simulink model "motor_cal"  (R2022b)
settings: Solver=FixedStepAuto  StartTime=0.0  StopTime=12  RelTol=1e-3  EnableMultiTasking=on
undefined symbols (not defined in the file or in its folder): ODR
libraries: raspberrypiBasiclib x6, raspberrypiIMUsensorslib x2, simulink x1
settings Model: Creator=sjohnson  LastModifiedBy=sjohnson
settings SolverCC: PositivePriorityOrder=on
settings OptimizationCC: EnhancedBackFolding=on  PassReuseOutputArgsAs=Individual arguments  ZeroExternalMemoryAtStartup=off  ZeroInternalMemoryAtStartup=off  MaxStackSize=64  OptimizeBlockOrder=speed  DifferentSizesBufferReuse=on  OptimizationCustomize=off  EfficientTunableParamExpr=on
settings DebuggingCC: ParameterTunabilityLossMsg=error
settings HardwareCC: ProdBitPerPointer=32  ProdBitPerSizeT=32  ProdBitPerPtrDiffT=32  ProdLargestAtomicInteger=Long  ProdLargestAtomicFloat=Double  ProdWordSize=32  ProdLongLongMode=on  ProdHWDeviceType=ARM Compatible->ARM Cortex  UseEmbeddedCoderFeatures=off  UseSimulinkCoderFeatures=off
settings ModelReferenceCC: UpdateModelReferenceTargets=AssumeUpToDate
settings RTWCC: Description=Embedded Coder  SystemTargetFile=ert.tlc  HardwareBoard=Raspberry Pi  TLCOptions="-aInlineSetEventsForThisBaseRateFcn=TLC_FALSE -aSuppressMultiTaskScheduler=TLC_FALSE  -aRateBasedStepFcn=0"  TemplateMakefile=ert_default_tmf  Toolchain=GNU GCC Embedded Linux  BuildConfiguration=Faster Runs
settings CodeAppCC: ForceParamTrailComments=on  IgnoreCustomStorageClasses=off  OperatorAnnotations=on  SimulinkDataObjDesc=on  SFDataObjDesc=on  MangleLength=10  InsertBlockDesc=on
settings ERTTargetCC: SupportNonInlinedSFcns=on  SupportVariableSizeSignals=on  ExtModeTransport=2  ExtModeStaticAlloc=on  ExtModeMexFile=ext_xcp  ExtModeIntrfLevel=Level2 - Open

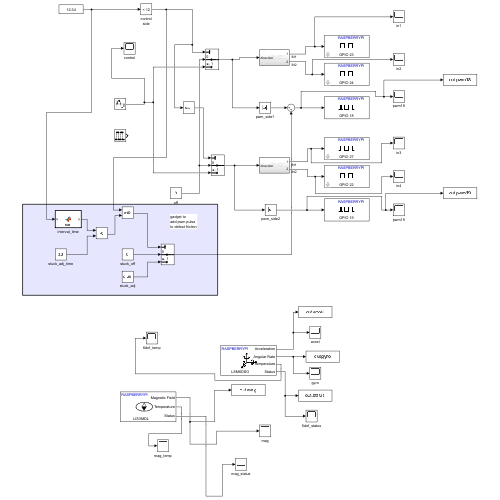
[thumbnail: Simulink's stored preview of the top-level diagram]
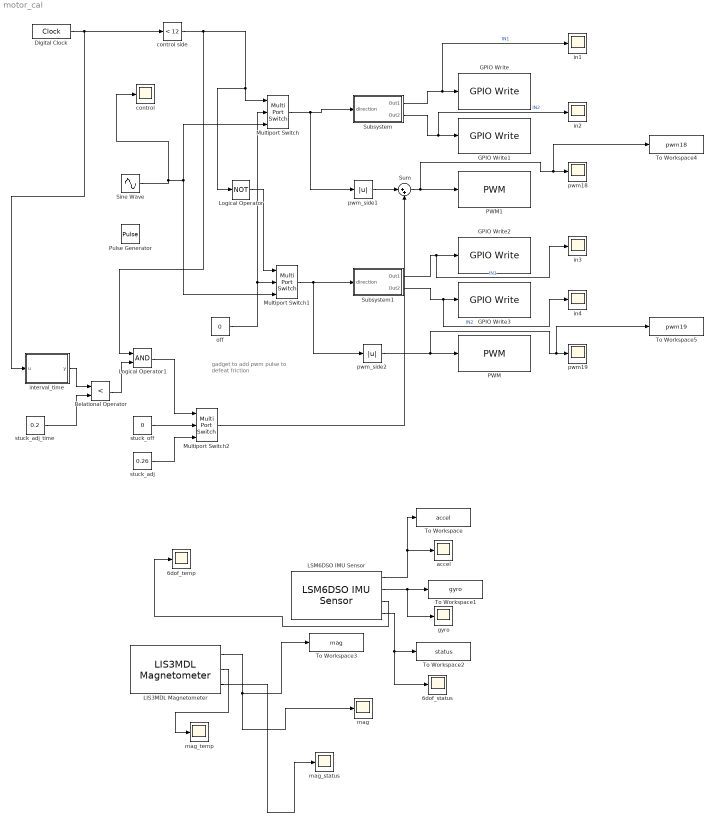
== system motor_cal ==
  note: gadget to
      | add pwm pulse
      | to defeat friction
  6dof_status : Scope
  6dof_temp : Scope
  Digital Clock : DigitalClock  SampleTime=.01
  GPIO Write : raspberrypiBasiclib/GPIO Write  board=Pi 4 Model B  gpio=23  direction=Output  blockPlatform=Raspberry Pi
  GPIO Write1 : raspberrypiBasiclib/GPIO Write  board=Pi 4 Model B  gpio=24  direction=Output  blockPlatform=Raspberry Pi
  GPIO Write2 : raspberrypiBasiclib/GPIO Write  board=Pi 4 Model B  gpio=27  direction=Output  blockPlatform=Raspberry Pi
  GPIO Write3 : raspberrypiBasiclib/GPIO Write  board=Pi 4 Model B  gpio=22  direction=Output  blockPlatform=Raspberry Pi
  LIS3MDL Magnetometer : raspberrypiIMUsensorslib/LIS3MDL Magnetometer  I2CModule=1  I2CAddress=0x1E  IsActiveMagnetometer=on  IsActiveTemperature=on  IsStatus=on  SampleTime=-1  MagnetometerRange=+/- 400 uT  MagnetometerODR=155 Hz
  LSM6DSO IMU Sensor : raspberrypiIMUsensorslib/LSM6DSO IMU Sensor  I2CModule=1  I2CAddress=0x6B  IsActiveAcceleration=on  IsActiveAngularRate=on  IsActiveTemperature=on  IsActiveStatus=on  IsActiveTimeStamp=off  SampleTime=-1  QueueSizeFactor=3  AccelerometerRange=+/- 2g  AccelerometerODR=104 Hz  AccelSelectCompositeFilter=No filter  AccelLPF2BW=ODR/4  AccelHPFBW=ODR/4  GyroscopeRange=125 dps  GyroscopeODR=104 Hz  EnableGyroHPF=off  GyroHPFBW=0.016 Hz  EnableGyroLPF=off  GyroLPFBWMode=0
  Logical Operator : Logic  Operator=NOT  Inputs=1  AllPortsSameDT=off  OutDataTypeStr=boolean
  Logical Operator1 : Logic  AllPortsSameDT=off  OutDataTypeStr=boolean
  Multiport Switch : MultiPortSwitch  DataPortOrder=Zero-based contiguous  Inputs=2  zeroidx=on  SaturateOnIntegerOverflow=off  InputSameDT=off
  Multiport Switch1 : MultiPortSwitch  DataPortOrder=Zero-based contiguous  Inputs=2  zeroidx=on  SaturateOnIntegerOverflow=off  InputSameDT=off
  Multiport Switch2 : MultiPortSwitch  DataPortOrder=Zero-based contiguous  Inputs=2  zeroidx=on  SaturateOnIntegerOverflow=off  InputSameDT=off
  PWM : raspberrypiBasiclib/PWM  board=Pi 4 Model B  Pin_=19  Frequency=50  blockPlatform=Raspberry Pi
  PWM1 : raspberrypiBasiclib/PWM  board=Pi 4 Model B  Pin_=18  Frequency=50  blockPlatform=Raspberry Pi
  Pulse Generator : DiscretePulseGenerator  Period=200  PulseWidth=50  SampleTime=0.01
  Relational Operator : RelationalOperator  Operator=<  OutDataTypeStr=boolean  RndMeth=Simplest  InputSameDT=off
  Sine Wave : Sin  Amplitude=0.4  Frequency=pi/3  SampleTime=0.01
  Subsystem : Subsystem
  Subsystem1 : Subsystem
  Sum : Sum  Inputs=|++
  To Workspace : ToWorkspace  VariableName=accel  SaveFormat=Structure With Time  SampleTime=-1
  To Workspace1 : ToWorkspace  VariableName=gyro  SaveFormat=Structure With Time  SampleTime=-1
  To Workspace2 : ToWorkspace  VariableName=status  SaveFormat=Structure With Time  SampleTime=-1
  To Workspace3 : ToWorkspace  VariableName=mag  SaveFormat=Structure With Time  SampleTime=-1
  To Workspace4 : ToWorkspace  VariableName=pwm18  SaveFormat=Structure With Time  SampleTime=-1
  To Workspace5 : ToWorkspace  VariableName=pwm19  SaveFormat=Structure With Time  SampleTime=-1
  accel : Scope
  control : Scope
  control side : simulink/Logic and Bit Operations/Compare To Constant  relop=<  const=12  OutDataTypeStr=boolean
  gyro : Scope
  in{1..4} (4 alike) : Scope
  interval_time : MATLAB Function  TreatAsAtomicUnit=on
  mag : Scope
  mag_status : Scope
  mag_temp : Scope
  off : Constant  Value=0
  pwm18 : Scope
  pwm19 : Scope
  pwm_side1 : Abs  SaturateOnIntegerOverflow=off
  pwm_side2 : Abs  SaturateOnIntegerOverflow=off
  stuck_adj : Constant  Value=0.26
  stuck_adj_time : Constant  Value=0.2
  stuck_off : Constant  Value=0
  wires:
  Subsystem/1(Out1) -> in1/1, GPIO Write/1  "IN1"
  Subsystem/2(Out2) -> in2/1, GPIO Write1/1  "IN2"
  Subsystem1/1(Out1) -> in3/1, GPIO Write2/1  "IN1"
  Subsystem1/2(Out2) -> in4/1, GPIO Write3/1  "IN2"
  Multiport Switch/1 -> pwm_side1/1, Subsystem/1(direction)
  control side/1 -> Logical Operator1/1, Logical Operator/1, Multiport Switch/1
  Multiport Switch1/1 -> pwm_side2/1, Subsystem1/1(direction)
  Logical Operator/1 -> Multiport Switch1/1
  Sine Wave/1 -> control/1, Multiport Switch1/3, Multiport Switch/3
  off/1 -> Multiport Switch/2, Multiport Switch1/2
  Sum/1 -> To Workspace4/1, pwm18/1, PWM1/1
  pwm_side2/1 -> PWM/1, To Workspace5/1, pwm19/1
  Digital Clock/1 -> interval_time/1(u), control side/1
  LIS3MDL Magnetometer/2 -> mag_temp/1
  LSM6DSO IMU Sensor/3 -> 6dof_temp/1
  LSM6DSO IMU Sensor/4 -> To Workspace2/1, 6dof_status/1
  LIS3MDL Magnetometer/1 -> To Workspace3/1, mag/1
  LSM6DSO IMU Sensor/1 -> accel/1, To Workspace/1
  LSM6DSO IMU Sensor/2 -> gyro/1, To Workspace1/1
  LIS3MDL Magnetometer/3 -> mag_status/1
  interval_time/1(y) -> Relational Operator/1
  stuck_adj_time/1 -> Relational Operator/2
  Logical Operator1/1 -> Multiport Switch2/1
  stuck_adj/1 -> Multiport Switch2/3
  stuck_off/1 -> Multiport Switch2/2
  pwm_side1/1 -> Sum/1
  Multiport Switch2/1 -> Sum/2
  Relational Operator/1 -> Logical Operator1/2

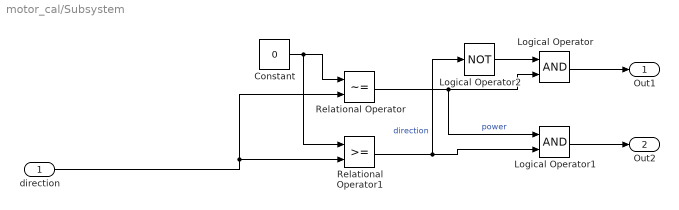
== system motor_cal/Subsystem ==
  direction : Inport
  Constant : Constant  Value=0
  Logical Operator : Logic  AllPortsSameDT=off  OutDataTypeStr=boolean
  Logical Operator1 : Logic  AllPortsSameDT=off  OutDataTypeStr=boolean
  Logical Operator2 : Logic  Operator=NOT  Inputs=1  AllPortsSameDT=off  OutDataTypeStr=boolean
  Relational Operator : RelationalOperator  Operator=~=  OutDataTypeStr=boolean  RndMeth=Simplest  InputSameDT=off
  Relational Operator1 : RelationalOperator  OutDataTypeStr=boolean  RndMeth=Simplest  InputSameDT=off
  Out1 : Outport
  Out2 : Outport  Port=2
  wires:
  Logical Operator/1 -> Out1/1
  Relational Operator1/1 -> Logical Operator2/1, Logical Operator1/2  "direction"
  Logical Operator1/1 -> Out2/1
  Logical Operator2/1 -> Logical Operator/1
  direction/1 -> Relational Operator/2, Relational Operator1/2
  Constant/1 -> Relational Operator1/1, Relational Operator/1
  Relational Operator/1 -> Logical Operator1/1, Logical Operator/2  "power"

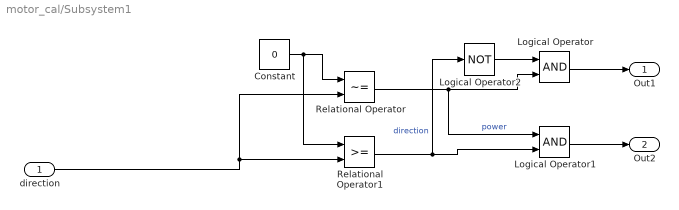
== system motor_cal/Subsystem1 ==
  direction : Inport
  Constant : Constant  Value=0
  Logical Operator : Logic  AllPortsSameDT=off  OutDataTypeStr=boolean
  Logical Operator1 : Logic  AllPortsSameDT=off  OutDataTypeStr=boolean
  Logical Operator2 : Logic  Operator=NOT  Inputs=1  AllPortsSameDT=off  OutDataTypeStr=boolean
  Relational Operator : RelationalOperator  Operator=~=  OutDataTypeStr=boolean  RndMeth=Simplest  InputSameDT=off
  Relational Operator1 : RelationalOperator  OutDataTypeStr=boolean  RndMeth=Simplest  InputSameDT=off
  Out1 : Outport
  Out2 : Outport  Port=2
  wires:
  Logical Operator/1 -> Out1/1
  Relational Operator1/1 -> Logical Operator2/1, Logical Operator1/2  "direction"
  Logical Operator1/1 -> Out2/1
  Logical Operator2/1 -> Logical Operator/1
  direction/1 -> Relational Operator/2, Relational Operator1/2
  Constant/1 -> Relational Operator1/1, Relational Operator/1
  Relational Operator/1 -> Logical Operator1/1, Logical Operator/2  "power"

== matlab function motor_cal/interval_time ==
  data: u input; y output
function y = fcn(u)

y = u - 3*floor(u/3);
